simulink model "MERGEBLOCK"  (R2021a)
settings: Solver=FixedStepDiscrete  StartTime=0.0  StopTime=10.0  RelTol=1e-3
libraries: simulink x1
settings Model: Creator=saurabh  LastModifiedBy=saurabh
settings SolverCC: AlgebraicLoopSolver=TrustRegion
settings DebuggingCC: SFMachineParentedDataDiag=warning
settings SFSimCC: CustomCodeUndefinedFunction=UseInterfaceOnly

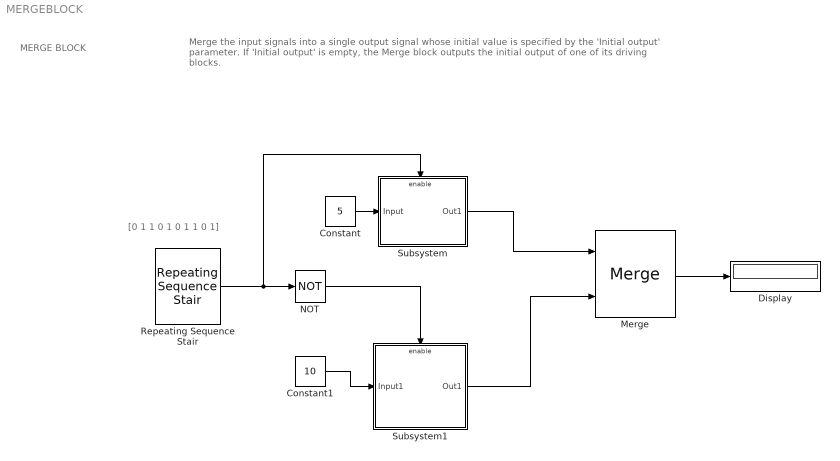
== system MERGEBLOCK ==
  note: Merge the input signals into a single output signal whose initial value is specified by the 'Initial output' parameter.
      | If 'Initial output' is empty, the Merge block outputs the initial output of one of its driving blocks.
  note: MERGE BLOCK
  note: [0 1 1 0 1 0 1 1 0 1]
  Constant : Constant  Value=5
  Constant1 : Constant  Value=10
  Display : Display
  Merge : Merge
  NOT : Logic  Operator=NOT  IconShape=distinctive  AllPortsSameDT=off  OutDataTypeStr=boolean
  Repeating Sequence Stair : simulink/Sources/Repeating Sequence Stair  OutValues=[0 1 1 0 1 0 1 1 0 1].'  tsamp=-1  OutMin=[]  OutMax=[]  OutDataTypeStr=double  OutputDataTypeScalingMode=double  OutDataType=fixdt(0,8)  ConRadixGroup=Best Precision: Vector-wise  OutScaling=2^-12
  Subsystem : Subsystem
  Subsystem1 : Subsystem
  wires:
  Subsystem/1(Out1) -> Merge/1
  Subsystem1/1(Out1) -> Merge/2
  Repeating Sequence Stair/1 -> Subsystem/Enable, NOT/1
  NOT/1 -> Subsystem1/Enable
  Merge/1 -> Display/1
  Constant/1 -> Subsystem/1(Input)
  Constant1/1 -> Subsystem1/1(Input1)

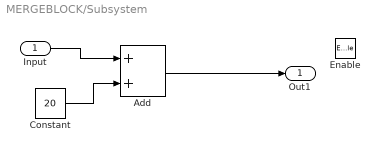
== system MERGEBLOCK/Subsystem ==
  Input : Inport
  Enable : EnablePort
  Add : Sum
  Constant : Constant  Value=20
  Out1 : Outport  VectorParamsAs1DForOutWhenUnconnected=off
  wires:
  Add/1 -> Out1/1
  Constant/1 -> Add/2
  Input/1 -> Add/1

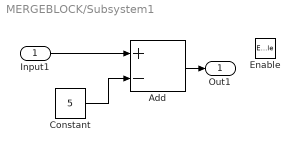
== system MERGEBLOCK/Subsystem1 ==
  Input1 : Inport
  Enable : EnablePort
  Add : Sum  Inputs=+-
  Constant : Constant  Value=5
  Out1 : Outport  VectorParamsAs1DForOutWhenUnconnected=off
  wires:
  Input1/1 -> Add/1
  Constant/1 -> Add/2
  Add/1 -> Out1/1
